simulink model "Motor"  (R2024a)
settings: Solver=FixedStepAuto  StartTime=0.0  StopTime=10  FixedStep=MotorSampleTime  RelTol=1e-3
model workspace (MAT data in the model file):
  MotorSampleTime = 0.001
undefined symbols (not defined in the file or in its folder): DiscIntNeverNeededParam
settings Model: SimulationMode=accelerator  Creator=17739  LastModifiedBy=17739

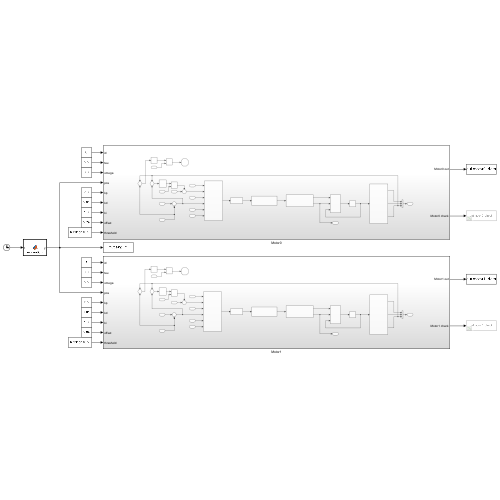
[thumbnail: Simulink's stored preview of the top-level diagram]
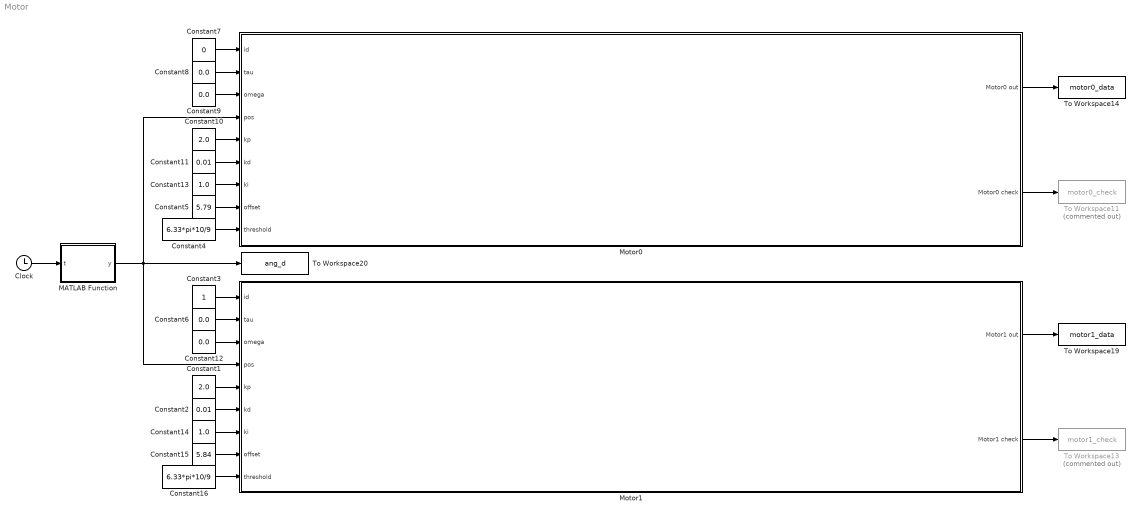
== system Motor ==
  Clock : Clock
  Constant1 : Constant  Value=2.0
  Constant10 : Constant  Value=2.0
  Constant11 : Constant  Value=0.01
  Constant{6,8..9,12} (4 alike) : Constant  Value=0.0
  Constant13 : Constant  Value=1.0
  Constant14 : Constant  Value=1.0
  Constant15 : Constant  Value=5.84
  Constant16 : Constant  Value=6.33*pi*10/9
  Constant2 : Constant  Value=0.01
  Constant3 : Constant
  Constant4 : Constant  Value=6.33*pi*10/9
  Constant5 : Constant  Value=5.79
  Constant7 : Constant  Value=0
  MATLAB Function : MATLAB Function  TreatAsAtomicUnit=on
  Motor0 : Subsystem
  Motor1 : Subsystem
  To Workspace11 : ToWorkspace  Commented=on  VariableName=motor0_check  SampleTime=-1
  To Workspace13 : ToWorkspace  Commented=on  VariableName=motor1_check  SampleTime=-1
  To Workspace14 : ToWorkspace  VariableName=motor0_data  SampleTime=-1
  To Workspace19 : ToWorkspace  VariableName=motor1_data  SampleTime=-1
  To Workspace20 : ToWorkspace  VariableName=ang_d  SampleTime=-1
  wires:
  Clock/1 -> MATLAB Function/1(t)
  Constant6/1 -> Motor1/2(tau)
  Constant15/1 -> Motor1/8(offset)
  Constant7/1 -> Motor0/1(id)
  Constant16/1 -> Motor1/9(threshold)
  Constant5/1 -> Motor0/8(offset)
  Constant13/1 -> Motor0/7(ki)
  Constant12/1 -> Motor1/3(omega)
  Constant4/1 -> Motor0/9(threshold)
  Constant9/1 -> Motor0/3(omega)
  Motor0/2(Motor0 check) -> To Workspace11/1
  Constant8/1 -> Motor0/2(tau)
  Constant11/1 -> Motor0/6(kd)
  Constant3/1 -> Motor1/1(id)
  Constant14/1 -> Motor1/7(ki)
  Motor1/2(Motor1 check) -> To Workspace13/1
  MATLAB Function/1(y) -> Motor0/4(pos), Motor1/4(pos), To Workspace20/1
  Constant2/1 -> Motor1/6(kd)
  Constant10/1 -> Motor0/5(kp)
  Constant1/1 -> Motor1/5(kp)
  Motor0/1(Motor0 out) -> To Workspace14/1
  Motor1/1(Motor1 out) -> To Workspace19/1

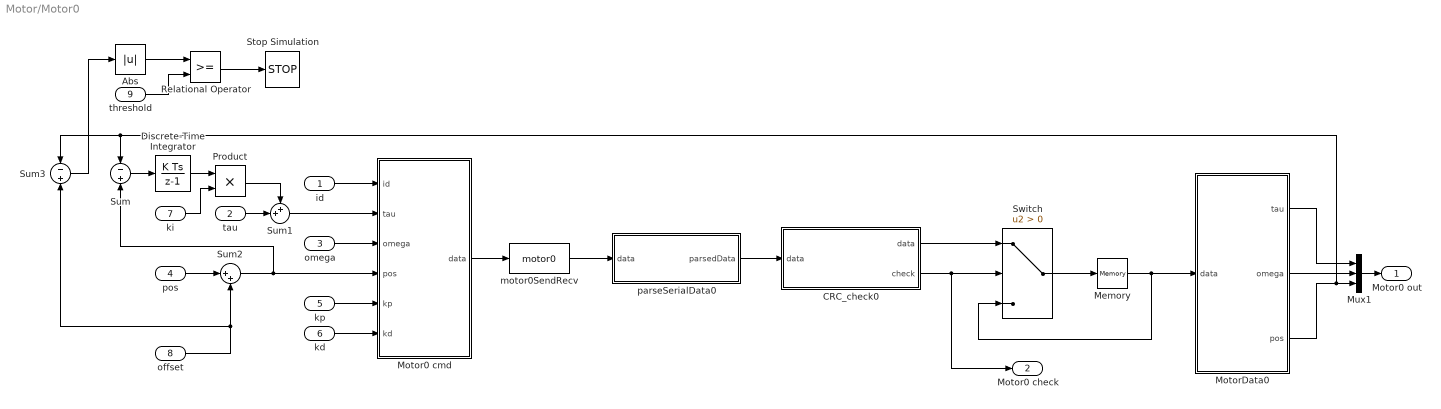
== system Motor/Motor0 ==
  id : Inport
  tau : Inport  Port=2
  omega : Inport  Port=3
  pos : Inport  Port=4
  kp : Inport  Port=5
  kd : Inport  Port=6
  ki : Inport  Port=7
  offset : Inport  Port=8
  threshold : Inport  Port=9
  Abs : Abs  SaturateOnIntegerOverflow=off
  CRC_check0 : MATLAB Function  TreatAsAtomicUnit=on
  Discrete-Time Integrator : DiscreteIntegrator  SampleTime=-1  ICPrevOutput=DiscIntNeverNeededParam  ICPrevScaledInput=DiscIntNeverNeededParam
  Memory : Memory  InheritSampleTime=on
  Motor0 cmd : MATLAB Function  TreatAsAtomicUnit=on
  MotorData0 : MATLAB Function  TreatAsAtomicUnit=on
  Mux1 : Mux  Inputs=3
  Product : Product
  Relational Operator : RelationalOperator  OutDataTypeStr=boolean  RndMeth=Simplest  InputSameDT=off
  Stop Simulation : Stop
  Sum : Sum  Inputs=-|+
  Sum1 : Sum  Inputs=++|
  Sum2 : Sum  Inputs=|++
  Sum3 : Sum  Inputs=-|+
  Switch : Switch  Criteria=u2 > Threshold  SaturateOnIntegerOverflow=off  InputSameDT=off
  motor0SendRecv : S-Function  FunctionName=motor0  SFunctionDeploymentMode=off  EnableBusSupport=off
  parseSerialData0 : MATLAB Function  TreatAsAtomicUnit=on
  Motor0 out : Outport
  Motor0 check : Outport  Port=2
  wires:
  MotorData0/2(omega) -> Mux1/2
  Motor0 cmd/1(data) -> motor0SendRecv/1
  parseSerialData0/1(parsedData) -> CRC_check0/1("data ")
  motor0SendRecv/1 -> parseSerialData0/1(data)
  Memory/1 -> MotorData0/1(data), Switch/3
  MotorData0/1(tau) -> Mux1/1
  Switch/1 -> Memory/1
  CRC_check0/1(data) -> Switch/1
  CRC_check0/2(check) -> Motor0 check/1, Switch/2
  Mux1/1 -> Motor0 out/1
  Sum3/1 -> Abs/1
  pos/1 -> Sum2/1
  Sum2/1 -> Motor0 cmd/4(pos), Sum/2
  Abs/1 -> Relational Operator/1
  Relational Operator/1 -> Stop Simulation/1
  offset/1 -> Sum3/2, Sum2/2
  Sum/1 -> Discrete-Time Integrator/1
  Product/1 -> Sum1/1
  Sum1/1 -> Motor0 cmd/2(tau)
  threshold/1 -> Relational Operator/2
  kd/1 -> Motor0 cmd/6(kd)
  Discrete-Time Integrator/1 -> Product/1
  tau/1 -> Sum1/2
  ki/1 -> Product/2
  MotorData0/3(pos) -> Sum3/1, Sum/1, Mux1/3
  omega/1 -> Motor0 cmd/3(omega)
  kp/1 -> Motor0 cmd/5(kp)
  id/1 -> Motor0 cmd/1(id)

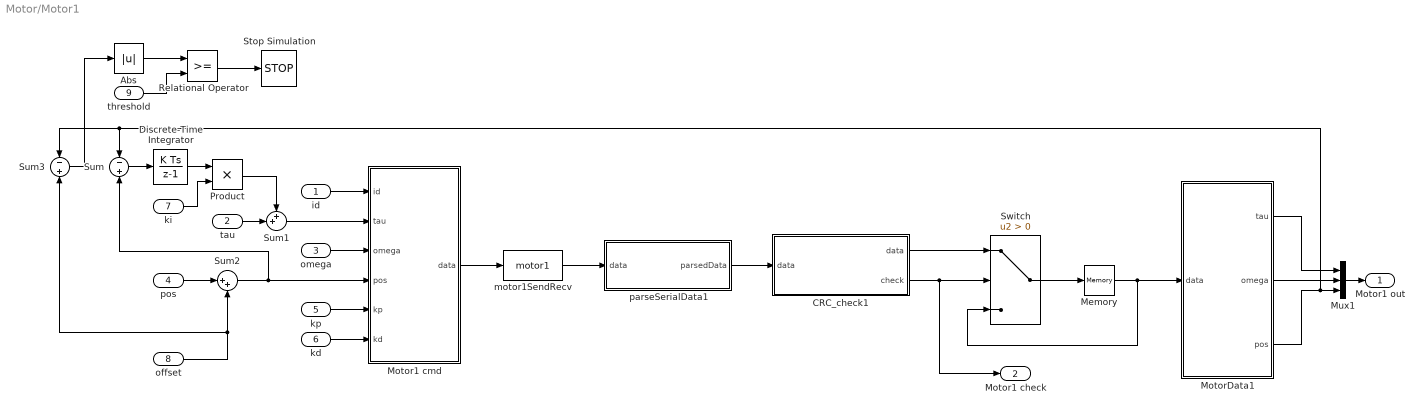
== system Motor/Motor1 ==
  id : Inport
  tau : Inport  Port=2
  omega : Inport  Port=3
  pos : Inport  Port=4
  kp : Inport  Port=5
  kd : Inport  Port=6
  ki : Inport  Port=7
  offset : Inport  Port=8
  threshold : Inport  Port=9
  Abs : Abs  SaturateOnIntegerOverflow=off
  CRC_check1 : MATLAB Function  TreatAsAtomicUnit=on
  Discrete-Time Integrator : DiscreteIntegrator  SampleTime=-1  ICPrevOutput=DiscIntNeverNeededParam  ICPrevScaledInput=DiscIntNeverNeededParam
  Memory : Memory  InheritSampleTime=on
  Motor1 cmd : MATLAB Function  TreatAsAtomicUnit=on
  MotorData1 : MATLAB Function  TreatAsAtomicUnit=on
  Mux1 : Mux  Inputs=3
  Product : Product
  Relational Operator : RelationalOperator  OutDataTypeStr=boolean  RndMeth=Simplest  InputSameDT=off
  Stop Simulation : Stop
  Sum : Sum  Inputs=-|+
  Sum1 : Sum  Inputs=++|
  Sum2 : Sum  Inputs=|++
  Sum3 : Sum  Inputs=-|+
  Switch : Switch  Criteria=u2 > Threshold  SaturateOnIntegerOverflow=off  InputSameDT=off
  motor1SendRecv : S-Function  FunctionName=motor1  SFunctionDeploymentMode=off  EnableBusSupport=off
  parseSerialData1 : MATLAB Function  TreatAsAtomicUnit=on
  Motor1 out : Outport
  Motor1 check : Outport  Port=2
  wires:
  MotorData1/2(omega) -> Mux1/2
  parseSerialData1/1(parsedData) -> CRC_check1/1("data ")
  motor1SendRecv/1 -> parseSerialData1/1(data)
  Memory/1 -> MotorData1/1(data), Switch/3
  MotorData1/1(tau) -> Mux1/1
  Switch/1 -> Memory/1
  CRC_check1/2(check) -> Motor1 check/1, Switch/2
  Mux1/1 -> Motor1 out/1
  CRC_check1/1(data) -> Switch/1
  Motor1 cmd/1(data) -> motor1SendRecv/1
  offset/1 -> Sum3/2, Sum2/2
  threshold/1 -> Relational Operator/2
  id/1 -> Motor1 cmd/1(id)
  Sum2/1 -> Sum/2, Motor1 cmd/4(pos)
  tau/1 -> Sum1/2
  ki/1 -> Product/2
  MotorData1/3(pos) -> Sum3/1, Sum/1, Mux1/3
  Discrete-Time Integrator/1 -> Product/1
  Abs/1 -> Relational Operator/1
  Relational Operator/1 -> Stop Simulation/1
  Product/1 -> Sum1/1
  pos/1 -> Sum2/1
  Sum3/1 -> Abs/1
  Sum/1 -> Discrete-Time Integrator/1
  kd/1 -> Motor1 cmd/6(kd)
  kp/1 -> Motor1 cmd/5(kp)
  omega/1 -> Motor1 cmd/3(omega)
  Sum1/1 -> Motor1 cmd/2(tau)

== matlab function Motor/Motor1/parseSerialData1 ==
  data: data input; parsedData output
function parsedData = parseSerialData(data)
    persistent buffer0;
    if isempty(buffer0)
        buffer0 = uint8([]);
    end

    % Append new data to buffer, ensuring data is a row vector
    buffer0 = [buffer0, data(:)']; 

    % Define header and data size
    header = uint8([253, 238]); % 定义包头
    dataSize = 16; % 你的数据包大小

    % Initialize parsedData as an empty uint8 array of size 16
    parsedData = uint8([253, 238, zeros(1, dataSize-2)]);

    % Check if the buffer contains a valid packet
    while length(buffer0) >= dataSize
        % Find the header in the buffer
        headerPos = findHeader(buffer0, header);

        % If header is found and there is enough data for a full packet
        if ~isempty(headerPos) && (headerPos(1) + dataSize - 1 <= length(buffer0))
            % Extract the valid packet
            for num = 1:dataSize
                parsedData(num) = buffer0(headerPos(1) + num - 1);
            end
            % Remove the extracted packet from the buffer
            if length(headerPos) > 1
                buffer0 = buffer0(headerPos(2):end);
            else
                buffer0 = buffer0((headerPos(1) + dataSize):end);
            end
            return; % Exit the function after finding the first valid packet
        else
            % If no valid packet is found, clear the buffer up to the header position
            if ~isempty(headerPos)
                buffer0 = buffer0(headerPos(1):end);
            else
                buffer0 = uint8([]);
            end
            break;
        end
    end
end

function pos = findHeader(buffer, header)
    pos = [];
    for i = 1:(length(buffer) - length(header) + 1)
        if all(buffer(i:i + length(header) - 1) == header)
            pos = i;
            return;
        end
    end
end

== matlab function Motor/MATLAB Function ==
  data: t input; y output
function y = motivation(t)
% f1 = 1; f2 = 0.75; f3 = 2/3; f4 = 0.5;% 频率成分
% if t >= 22
%     y = 6.33*pi*sin(2*pi*f1*(t-22));
% elseif t >= 14
%     y = 6.33*pi*sin(2*pi*f2*(t-14));
% elseif t >= 8
%     y = 6.33*pi*sin(2*pi*f3*(t-8));
% else
%     y = 6.33*pi*sin(2*pi*f4*t);
% end
y = 6.33*pi*sin(1.5*pi*t);
end

== matlab function Motor/Motor0/CRC_check0 ==
  data: data output size=[1 16]; check output; data input
function [data, check] = CRC_Check(data)

crc_ccitt_table = [
    0x0000, 0x1189, 0x2312, 0x329b, 0x4624, 0x57ad, 0x6536, 0x74bf, ...
    0x8c48, 0x9dc1, 0xaf5a, 0xbed3, 0xca6c, 0xdbe5, 0xe97e, 0xf8f7, ...
    0x1081, 0x0108, 0x3393, 0x221a, 0x56a5, 0x472c, 0x75b7, 0x643e, ...
    0x9cc9, 0x8d40, 0xbfdb, 0xae52, 0xdaed, 0xcb64, 0xf9ff, 0xe876, ...
    0x2102, 0x308b, 0x0210, 0x1399, 0x6726, 0x76af, 0x4434, 0x55bd, ...
    0xad4a, 0xbcc3, 0x8e58, 0x9fd1, 0xeb6e, 0xfae7, 0xc87c, 0xd9f5, ...
    0x3183, 0x200a, 0x1291, 0x0318, 0x77a7, 0x662e, 0x54b5, 0x453c, ...
    0xbdcb, 0xac42, 0x9ed9, 0x8f50, 0xfbef, 0xea66, 0xd8fd, 0xc974, ...
    0x4204, 0x538d, 0x6116, 0x709f, 0x0420, 0x15a9, 0x2732, 0x36bb, ...
    0xce4c, 0xdfc5, 0xed5e, 0xfcd7, 0x8868, 0x99e1, 0xab7a, 0xbaf3, ...
    0x5285, 0x430c, 0x7197, 0x601e, 0x14a1, 0x0528, 0x37b3, 0x263a, ...
    0xdecd, 0xcf44, 0xfddf, 0xec56, 0x98e9, 0x8960, 0xbbfb, 0xaa72, ...
    0x6306, 0x728f, 0x4014, 0x519d, 0x2522, 0x34ab, 0x0630, 0x17b9, ...
    0xef4e, 0xfec7, 0xcc5c, 0xddd5, 0xa96a, 0xb8e3, 0x8a78, 0x9bf1, ...
    0x7387, 0x620e, 0x5095, 0x411c, 0x35a3, 0x242a, 0x16b1, 0x0738, ...
    0xffcf, 0xee46, 0xdcdd, 0xcd54, 0xb9eb, 0xa862, 0x9af9, 0x8b70, ...
    0x8408, 0x9581, 0xa71a, 0xb693, 0xc22c, 0xd3a5, 0xe13e, 0xf0b7, ...
    0x0840, 0x19c9, 0x2b52, 0x3adb, 0x4e64, 0x5fed, 0x6d76, 0x7cff, ...
    0x9489, 0x8500, 0xb79b, 0xa612, 0xd2ad, 0xc324, 0xf1bf, 0xe036, ...
    0x18c1, 0x0948, 0x3bd3, 0x2a5a, 0x5ee5, 0x4f6c, 0x7df7, 0x6c7e, ...
    0xa50a, 0xb483, 0x8618, 0x9791, 0xe32e, 0xf2a7, 0xc03c, 0xd1b5, ...
    0x2942, 0x38cb, 0x0a50, 0x1bd9, 0x6f66, 0x7eef, 0x4c74, 0x5dfd, ...
    0xb58b, 0xa402, 0x9699, 0x8710, 0xf3af, 0xe226, 0xd0bd, 0xc134, ...
    0x39c3, 0x284a, 0x1ad1, 0x0b58, 0x7fe7, 0x6e6e, 0x5cf5, 0x4d7c, ...
    0xc60c, 0xd785, 0xe51e, 0xf497, 0x8028, 0x91a1, 0xa33a, 0xb2b3, ...
    0x4a44, 0x5bcd, 0x6956, 0x78df, 0x0c60, 0x1de9, 0x2f72, 0x3efb, ...
    0xd68d, 0xc704, 0xf59f, 0xe416, 0x90a9, 0x8120, 0xb3bb, 0xa232, ...
    0x5ac5, 0x4b4c, 0x79d7, 0x685e, 0x1ce1, 0x0d68, 0x3ff3, 0x2e7a, ...
    0xe70e, 0xf687, 0xc41c, 0xd595, 0xa12a, 0xb0a3, 0x8238, 0x93b1, ...
    0x6b46, 0x7acf, 0x4854, 0x59dd, 0x2d62, 0x3ceb, 0x0e70, 0x1ff9, ...
    0xf78f, 0xe606, 0xd49d, 0xc514, 0xb1ab, 0xa022, 0x92b9, 0x8330, ...
    0x7bc7, 0x6a4e, 0x58d5, 0x495c, 0x3de3, 0x2c6a, 0x1ef1, 0x0f78 ...
    ];

crc = uint16(0);
for i = 1:14
    tableIndex = bitand(bitxor(crc, uint16(data(i))), uint16(0xff));
    crc = bitxor(bitshift(crc, -8), crc_ccitt_table(tableIndex + 1));
end
check = false;
if typecast(uint8(data(end-1:end)), 'uint16') == crc
    check = true;
end
end

== matlab function Motor/Motor0/Motor0 cmd ==
  data: id input; data output size=[1 17]; tau input; omega input; pos input; kp input; kd input
function data = MotorCmd(id, tau, omega, pos, kp, kd)
data = uint8([hex2dec('FE'), hex2dec('EE'), ...
    16 + id, ...
    typecast(int16(fix(tau * 256)), 'uint8'), ...
    typecast(int16(fix(omega / (2 * pi) * 256)), 'uint8'), ...
    typecast(int32(fix(pos / (2 * pi) * 32768)), 'uint8'), ...
    typecast(int16(fix(kp * 1280)), 'uint8'), ...
    typecast(int16(fix(kd * 1280)), 'uint8'), ...
    0, 0]); % CRC16 计算稍后添加

% 计算并添加 CRC16 校验
crc = calculateCRC(data(1:15)); % 自定义 CRC 计算函数
data(16:17) = typecast(uint16(crc), 'uint8');
end
% 自定义 CRC 计算函数
function crc = calculateCRC(data)
crc_ccitt_table = [
    0x0000, 0x1189, 0x2312, 0x329b, 0x4624, 0x57ad, 0x6536, 0x74bf, ...
    0x8c48, 0x9dc1, 0xaf5a, 0xbed3, 0xca6c, 0xdbe5, 0xe97e, 0xf8f7, ...
    0x1081, 0x0108, 0x3393, 0x221a, 0x56a5, 0x472c, 0x75b7, 0x643e, ...
    0x9cc9, 0x8d40, 0xbfdb, 0xae52, 0xdaed, 0xcb64, 0xf9ff, 0xe876, ...
    0x2102, 0x308b, 0x0210, 0x1399, 0x6726, 0x76af, 0x4434, 0x55bd, ...
    0xad4a, 0xbcc3, 0x8e58, 0x9fd1, 0xeb6e, 0xfae7, 0xc87c, 0xd9f5, ...
    0x3183, 0x200a, 0x1291, 0x0318, 0x77a7, 0x662e, 0x54b5, 0x453c, ...
    0xbdcb, 0xac42, 0x9ed9, 0x8f50, 0xfbef, 0xea66, 0xd8fd, 0xc974, ...
    0x4204, 0x538d, 0x6116, 0x709f, 0x0420, 0x15a9, 0x2732, 0x36bb, ...
    0xce4c, 0xdfc5, 0xed5e, 0xfcd7, 0x8868, 0x99e1, 0xab7a, 0xbaf3, ...
    0x5285, 0x430c, 0x7197, 0x601e, 0x14a1, 0x0528, 0x37b3, 0x263a, ...
    0xdecd, 0xcf44, 0xfddf, 0xec56, 0x98e9, 0x8960, 0xbbfb, 0xaa72, ...
    0x6306, 0x728f, 0x4014, 0x519d, 0x2522, 0x34ab, 0x0630, 0x17b9, ...
    0xef4e, 0xfec7, 0xcc5c, 0xddd5, 0xa96a, 0xb8e3, 0x8a78, 0x9bf1, ...
    0x7387, 0x620e, 0x5095, 0x411c, 0x35a3, 0x242a, 0x16b1, 0x0738, ...
    0xffcf, 0xee46, 0xdcdd, 0xcd54, 0xb9eb, 0xa862, 0x9af9, 0x8b70, ...
    0x8408, 0x9581, 0xa71a, 0xb693, 0xc22c, 0xd3a5, 0xe13e, 0xf0b7, ...
    0x0840, 0x19c9, 0x2b52, 0x3adb, 0x4e64, 0x5fed, 0x6d76, 0x7cff, ...
    0x9489, 0x8500, 0xb79b, 0xa612, 0xd2ad, 0xc324, 0xf1bf, 0xe036, ...
    0x18c1, 0x0948, 0x3bd3, 0x2a5a, 0x5ee5, 0x4f6c, 0x7df7, 0x6c7e, ...
    0xa50a, 0xb483, 0x8618, 0x9791, 0xe32e, 0xf2a7, 0xc03c, 0xd1b5, ...
    0x2942, 0x38cb, 0x0a50, 0x1bd9, 0x6f66, 0x7eef, 0x4c74, 0x5dfd, ...
    0xb58b, 0xa402, 0x9699, 0x8710, 0xf3af, 0xe226, 0xd0bd, 0xc134, ...
    0x39c3, 0x284a, 0x1ad1, 0x0b58, 0x7fe7, 0x6e6e, 0x5cf5, 0x4d7c, ...
    0xc60c, 0xd785, 0xe51e, 0xf497, 0x8028, 0x91a1, 0xa33a, 0xb2b3, ...
    0x4a44, 0x5bcd, 0x6956, 0x78df, 0x0c60, 0x1de9, 0x2f72, 0x3efb, ...
    0xd68d, 0xc704, 0xf59f, 0xe416, 0x90a9, 0x8120, 0xb3bb, 0xa232, ...
    0x5ac5, 0x4b4c, 0x79d7, 0x685e, 0x1ce1, 0x0d68, 0x3ff3, 0x2e7a, ...
    0xe70e, 0xf687, 0xc41c, 0xd595, 0xa12a, 0xb0a3, 0x8238, 0x93b1, ...
    0x6b46, 0x7acf, 0x4854, 0x59dd, 0x2d62, 0x3ceb, 0x0e70, 0x1ff9, ...
    0xf78f, 0xe606, 0xd49d, 0xc514, 0xb1ab, 0xa022, 0x92b9, 0x8330, ...
    0x7bc7, 0x6a4e, 0x58d5, 0x495c, 0x3de3, 0x2c6a, 0x1ef1, 0x0f78 ...
    ];

crc = uint16(0);
for i = 1:length(data)
    tableIndex = bitand(bitxor(crc, uint16(data(i))), uint16(0xff));
    crc = bitxor(bitshift(crc, -8), crc_ccitt_table(tableIndex + 1));
end
end

== matlab function Motor/Motor0/MotorData0 ==
  data: data input; tau output size=1; omega output size=1; pos output size=1
function [tau, omega, pos] = MotorData(data)
tau = double(typecast(uint8(data(4:5)), 'int16')) / 256;
omega = double(typecast(uint8(data(6:7)), 'int16')) / 256 * 2 * pi;
pos = double(typecast(uint8(data(8:11)), 'int32')) / 32768 * 2 * pi;
end

== matlab function Motor/Motor0/parseSerialData0 ==
  data: data input; parsedData output
function parsedData = parseSerialData(data)
persistent buffer0;
if isempty(buffer0)
    buffer0 = uint8([]);
end

% Append new data to buffer, ensuring data is a row vector
buffer0 = [buffer0, data(:)'];

% Define header and data size
header = uint8([253, 238]); % 定义包头
dataSize = 16; % 你的数据包大小

% Initialize parsedData as an empty uint8 array of size 16
parsedData = uint8([253, 238, zeros(1, dataSize-2)]);

% Check if the buffer contains a valid packet
while length(buffer0) >= dataSize
    % Find the header in the buffer
    headerPos = findHeader(buffer0, header);

    % If header is found and there is enough data for a full packet
    if ~isempty(headerPos) && (headerPos(1) + dataSize - 1 <= length(buffer0))
        % Extract the valid packet
        for num = 1:dataSize
            parsedData(num) = buffer0(headerPos(1) + num - 1);
        end
        % Remove the extracted packet from the buffer
        if length(headerPos) > 1
            buffer0 = buffer0(headerPos(2):end);
        else
            buffer0 = buffer0((headerPos(1) + dataSize):end);
        end
        return; % Exit the function after finding the first valid packet
    else
        % If no valid packet is found, clear the buffer up to the header position
        if ~isempty(headerPos)
            buffer0 = buffer0(headerPos(1):end);
        else
            buffer0 = uint8([]);
        end
        break;
    end
end
end

function pos = findHeader(buffer, header)
pos = [];
for i = 1:(length(buffer) - length(header) + 1)
    if all(buffer(i:i + length(header) - 1) == header)
        pos = i;
        return;
    end
end
end

== matlab function Motor/Motor1/CRC_check1 ==
  data: data output size=[1 16]; check output; data input
function [data, check] = CRC_Check(data)

crc_ccitt_table = [
    0x0000, 0x1189, 0x2312, 0x329b, 0x4624, 0x57ad, 0x6536, 0x74bf, ...
    0x8c48, 0x9dc1, 0xaf5a, 0xbed3, 0xca6c, 0xdbe5, 0xe97e, 0xf8f7, ...
    0x1081, 0x0108, 0x3393, 0x221a, 0x56a5, 0x472c, 0x75b7, 0x643e, ...
    0x9cc9, 0x8d40, 0xbfdb, 0xae52, 0xdaed, 0xcb64, 0xf9ff, 0xe876, ...
    0x2102, 0x308b, 0x0210, 0x1399, 0x6726, 0x76af, 0x4434, 0x55bd, ...
    0xad4a, 0xbcc3, 0x8e58, 0x9fd1, 0xeb6e, 0xfae7, 0xc87c, 0xd9f5, ...
    0x3183, 0x200a, 0x1291, 0x0318, 0x77a7, 0x662e, 0x54b5, 0x453c, ...
    0xbdcb, 0xac42, 0x9ed9, 0x8f50, 0xfbef, 0xea66, 0xd8fd, 0xc974, ...
    0x4204, 0x538d, 0x6116, 0x709f, 0x0420, 0x15a9, 0x2732, 0x36bb, ...
    0xce4c, 0xdfc5, 0xed5e, 0xfcd7, 0x8868, 0x99e1, 0xab7a, 0xbaf3, ...
    0x5285, 0x430c, 0x7197, 0x601e, 0x14a1, 0x0528, 0x37b3, 0x263a, ...
    0xdecd, 0xcf44, 0xfddf, 0xec56, 0x98e9, 0x8960, 0xbbfb, 0xaa72, ...
    0x6306, 0x728f, 0x4014, 0x519d, 0x2522, 0x34ab, 0x0630, 0x17b9, ...
    0xef4e, 0xfec7, 0xcc5c, 0xddd5, 0xa96a, 0xb8e3, 0x8a78, 0x9bf1, ...
    0x7387, 0x620e, 0x5095, 0x411c, 0x35a3, 0x242a, 0x16b1, 0x0738, ...
    0xffcf, 0xee46, 0xdcdd, 0xcd54, 0xb9eb, 0xa862, 0x9af9, 0x8b70, ...
    0x8408, 0x9581, 0xa71a, 0xb693, 0xc22c, 0xd3a5, 0xe13e, 0xf0b7, ...
    0x0840, 0x19c9, 0x2b52, 0x3adb, 0x4e64, 0x5fed, 0x6d76, 0x7cff, ...
    0x9489, 0x8500, 0xb79b, 0xa612, 0xd2ad, 0xc324, 0xf1bf, 0xe036, ...
    0x18c1, 0x0948, 0x3bd3, 0x2a5a, 0x5ee5, 0x4f6c, 0x7df7, 0x6c7e, ...
    0xa50a, 0xb483, 0x8618, 0x9791, 0xe32e, 0xf2a7, 0xc03c, 0xd1b5, ...
    0x2942, 0x38cb, 0x0a50, 0x1bd9, 0x6f66, 0x7eef, 0x4c74, 0x5dfd, ...
    0xb58b, 0xa402, 0x9699, 0x8710, 0xf3af, 0xe226, 0xd0bd, 0xc134, ...
    0x39c3, 0x284a, 0x1ad1, 0x0b58, 0x7fe7, 0x6e6e, 0x5cf5, 0x4d7c, ...
    0xc60c, 0xd785, 0xe51e, 0xf497, 0x8028, 0x91a1, 0xa33a, 0xb2b3, ...
    0x4a44, 0x5bcd, 0x6956, 0x78df, 0x0c60, 0x1de9, 0x2f72, 0x3efb, ...
    0xd68d, 0xc704, 0xf59f, 0xe416, 0x90a9, 0x8120, 0xb3bb, 0xa232, ...
    0x5ac5, 0x4b4c, 0x79d7, 0x685e, 0x1ce1, 0x0d68, 0x3ff3, 0x2e7a, ...
    0xe70e, 0xf687, 0xc41c, 0xd595, 0xa12a, 0xb0a3, 0x8238, 0x93b1, ...
    0x6b46, 0x7acf, 0x4854, 0x59dd, 0x2d62, 0x3ceb, 0x0e70, 0x1ff9, ...
    0xf78f, 0xe606, 0xd49d, 0xc514, 0xb1ab, 0xa022, 0x92b9, 0x8330, ...
    0x7bc7, 0x6a4e, 0x58d5, 0x495c, 0x3de3, 0x2c6a, 0x1ef1, 0x0f78 ...
    ];

crc = uint16(0);
for i = 1:14
    tableIndex = bitand(bitxor(crc, uint16(data(i))), uint16(0xff));
    crc = bitxor(bitshift(crc, -8), crc_ccitt_table(tableIndex + 1));
end
check = false;
if typecast(uint8(data(end-1:end)), 'uint16') == crc
    check = true;
end
end

== matlab function Motor/Motor1/Motor1 cmd ==
  data: data output size=[1 17]; id input; tau input; omega input; pos input; kp input; kd input
function data = MotorCmd(id, tau, omega, pos, kp, kd)
data = uint8([hex2dec('FE'), hex2dec('EE'), ...
    16 + id, ...
    typecast(int16(fix(tau * 256)), 'uint8'), ...
    typecast(int16(fix(omega / (2 * pi) * 256)), 'uint8'), ...
    typecast(int32(fix(pos / (2 * pi) * 32768)), 'uint8'), ...
    typecast(int16(fix(kp * 1280)), 'uint8'), ...
    typecast(int16(fix(kd * 1280)), 'uint8'), ...
    0, 0]); % CRC16 计算稍后添加

% 计算并添加 CRC16 校验
crc = calculateCRC(data(1:15)); % 自定义 CRC 计算函数
data(16:17) = typecast(uint16(crc), 'uint8');
end
% 自定义 CRC 计算函数
function crc = calculateCRC(data)
crc_ccitt_table = [
    0x0000, 0x1189, 0x2312, 0x329b, 0x4624, 0x57ad, 0x6536, 0x74bf, ...
    0x8c48, 0x9dc1, 0xaf5a, 0xbed3, 0xca6c, 0xdbe5, 0xe97e, 0xf8f7, ...
    0x1081, 0x0108, 0x3393, 0x221a, 0x56a5, 0x472c, 0x75b7, 0x643e, ...
    0x9cc9, 0x8d40, 0xbfdb, 0xae52, 0xdaed, 0xcb64, 0xf9ff, 0xe876, ...
    0x2102, 0x308b, 0x0210, 0x1399, 0x6726, 0x76af, 0x4434, 0x55bd, ...
    0xad4a, 0xbcc3, 0x8e58, 0x9fd1, 0xeb6e, 0xfae7, 0xc87c, 0xd9f5, ...
    0x3183, 0x200a, 0x1291, 0x0318, 0x77a7, 0x662e, 0x54b5, 0x453c, ...
    0xbdcb, 0xac42, 0x9ed9, 0x8f50, 0xfbef, 0xea66, 0xd8fd, 0xc974, ...
    0x4204, 0x538d, 0x6116, 0x709f, 0x0420, 0x15a9, 0x2732, 0x36bb, ...
    0xce4c, 0xdfc5, 0xed5e, 0xfcd7, 0x8868, 0x99e1, 0xab7a, 0xbaf3, ...
    0x5285, 0x430c, 0x7197, 0x601e, 0x14a1, 0x0528, 0x37b3, 0x263a, ...
    0xdecd, 0xcf44, 0xfddf, 0xec56, 0x98e9, 0x8960, 0xbbfb, 0xaa72, ...
    0x6306, 0x728f, 0x4014, 0x519d, 0x2522, 0x34ab, 0x0630, 0x17b9, ...
    0xef4e, 0xfec7, 0xcc5c, 0xddd5, 0xa96a, 0xb8e3, 0x8a78, 0x9bf1, ...
    0x7387, 0x620e, 0x5095, 0x411c, 0x35a3, 0x242a, 0x16b1, 0x0738, ...
    0xffcf, 0xee46, 0xdcdd, 0xcd54, 0xb9eb, 0xa862, 0x9af9, 0x8b70, ...
    0x8408, 0x9581, 0xa71a, 0xb693, 0xc22c, 0xd3a5, 0xe13e, 0xf0b7, ...
    0x0840, 0x19c9, 0x2b52, 0x3adb, 0x4e64, 0x5fed, 0x6d76, 0x7cff, ...
    0x9489, 0x8500, 0xb79b, 0xa612, 0xd2ad, 0xc324, 0xf1bf, 0xe036, ...
    0x18c1, 0x0948, 0x3bd3, 0x2a5a, 0x5ee5, 0x4f6c, 0x7df7, 0x6c7e, ...
    0xa50a, 0xb483, 0x8618, 0x9791, 0xe32e, 0xf2a7, 0xc03c, 0xd1b5, ...
    0x2942, 0x38cb, 0x0a50, 0x1bd9, 0x6f66, 0x7eef, 0x4c74, 0x5dfd, ...
    0xb58b, 0xa402, 0x9699, 0x8710, 0xf3af, 0xe226, 0xd0bd, 0xc134, ...
    0x39c3, 0x284a, 0x1ad1, 0x0b58, 0x7fe7, 0x6e6e, 0x5cf5, 0x4d7c, ...
    0xc60c, 0xd785, 0xe51e, 0xf497, 0x8028, 0x91a1, 0xa33a, 0xb2b3, ...
    0x4a44, 0x5bcd, 0x6956, 0x78df, 0x0c60, 0x1de9, 0x2f72, 0x3efb, ...
    0xd68d, 0xc704, 0xf59f, 0xe416, 0x90a9, 0x8120, 0xb3bb, 0xa232, ...
    0x5ac5, 0x4b4c, 0x79d7, 0x685e, 0x1ce1, 0x0d68, 0x3ff3, 0x2e7a, ...
    0xe70e, 0xf687, 0xc41c, 0xd595, 0xa12a, 0xb0a3, 0x8238, 0x93b1, ...
    0x6b46, 0x7acf, 0x4854, 0x59dd, 0x2d62, 0x3ceb, 0x0e70, 0x1ff9, ...
    0xf78f, 0xe606, 0xd49d, 0xc514, 0xb1ab, 0xa022, 0x92b9, 0x8330, ...
    0x7bc7, 0x6a4e, 0x58d5, 0x495c, 0x3de3, 0x2c6a, 0x1ef1, 0x0f78 ...
    ];

crc = uint16(0);
for i = 1:length(data)
    tableIndex = bitand(bitxor(crc, uint16(data(i))), uint16(0xff));
    crc = bitxor(bitshift(crc, -8), crc_ccitt_table(tableIndex + 1));
end
end

== matlab function Motor/Motor1/MotorData1 ==
  data: data input; tau output size=1; omega output size=1; pos output size=1
function [tau, omega, pos] = MotorData(data)
tau = double(typecast(uint8(data(4:5)), 'int16')) / 256;
omega = double(typecast(uint8(data(6:7)), 'int16')) / 256 * 2 * pi;
pos = double(typecast(uint8(data(8:11)), 'int32')) / 32768 * 2 * pi;
end
